simulink model "waffle_kin_sim"  (R2020a)
settings: Solver=FixedStepAuto  StartTime=0.0  StopTime=inf  FixedStep=1e-4  RelTol=1e-3
model workspace (MAT data in the model file):
  d = 0.288
  r = 0.033
undefined symbols (not defined in the file): X, Y
libraries: robotlib x11

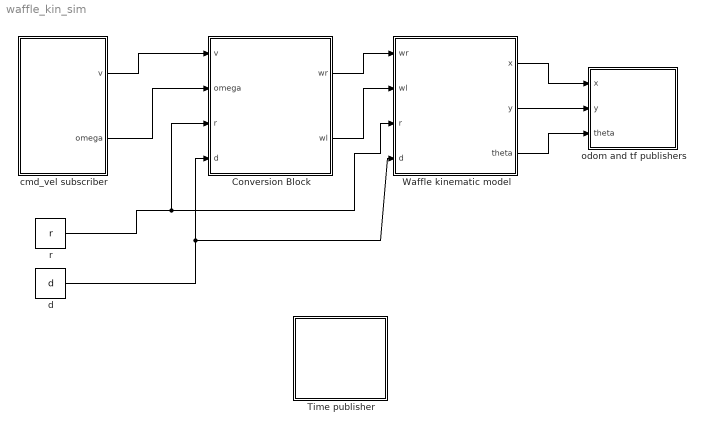
== system waffle_kin_sim ==
  Conversion Block : Subsystem  mask{state0=[0,0,0,0]}
      mask prompts: state0 "Initial conditions (x0, y0, theta0)"
  Time publisher : Subsystem
  Waffle kinematic model : Subsystem  mask{state0=[0,0,0]}
      mask prompts: state0 "Initial conditions (x0, y0, theta0)"
  cmd_vel subscriber : Subsystem
  d : Constant  Value=d
  odom and tf publishers : Subsystem  mask{simPublishRate=100}
      mask prompts: simPublishRate "Publising rate [Hz]"
  r : Constant  Value=r
  wires:
  Waffle kinematic model/1(x) -> odom and tf publishers/1(x)
  Waffle kinematic model/2(y) -> odom and tf publishers/2(y)
  Waffle kinematic model/3(theta) -> odom and tf publishers/3(theta)
  cmd_vel subscriber/1(v) -> Conversion Block/1(v)
  cmd_vel subscriber/2(omega) -> Conversion Block/2(omega)
  Conversion Block/1(wr) -> Waffle kinematic model/1(wr)
  Conversion Block/2(wl) -> Waffle kinematic model/2(wl)
  d/1 -> Conversion Block/4(d), Waffle kinematic model/4(d)
  r/1 -> Waffle kinematic model/3(r), Conversion Block/3(r)

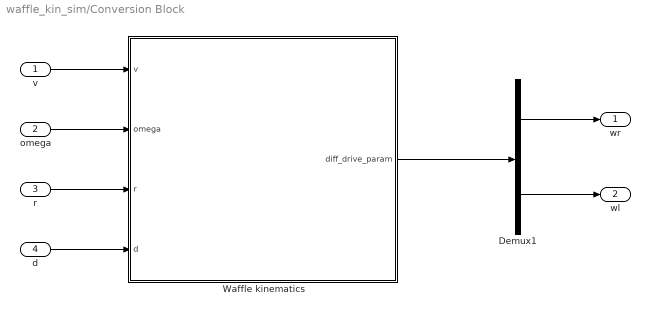
== system waffle_kin_sim/Conversion Block ==
  v : Inport
  omega : Inport  Port=2
  r : Inport  Port=3
  d : Inport  Port=4
  Demux1 : Demux  Outputs=2
  Waffle kinematics : MATLAB Function  TreatAsAtomicUnit=on
  wr : Outport  VectorParamsAs1DForOutWhenUnconnected=off
  wl : Outport  Port=2  VectorParamsAs1DForOutWhenUnconnected=off
  wires:
  Demux1/2 -> wl/1
  Demux1/1 -> wr/1
  d/1 -> Waffle kinematics/4(d)
  r/1 -> Waffle kinematics/3(r)
  v/1 -> Waffle kinematics/1(v)
  Waffle kinematics/1(diff_drive_param) -> Demux1/1
  omega/1 -> Waffle kinematics/2(omega)

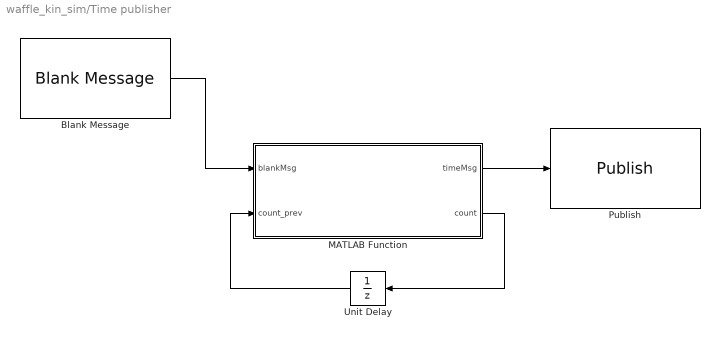
== system waffle_kin_sim/Time publisher ==
  Blank Message : robotlib/Blank Message  messageClass=Message  entityType=rosgraph_msgs/Clock  messageType=rosgraph_msgs/Clock  SampleTime=1e-4
  MATLAB Function : MATLAB Function  TreatAsAtomicUnit=on
  Publish : robotlib/Publish  topicSource=Specify your own  topic=/clock  messageType=rosgraph_msgs/Clock  messageQueueLength=1
  Unit Delay : UnitDelay  SampleTime=1e-4  HasFrameUpgradeWarning=on
  wires:
  MATLAB Function/1(timeMsg) -> Publish/1
  Blank Message/1 -> MATLAB Function/1(blankMsg)
  MATLAB Function/2(count) -> Unit Delay/1
  Unit Delay/1 -> MATLAB Function/2(count_prev)

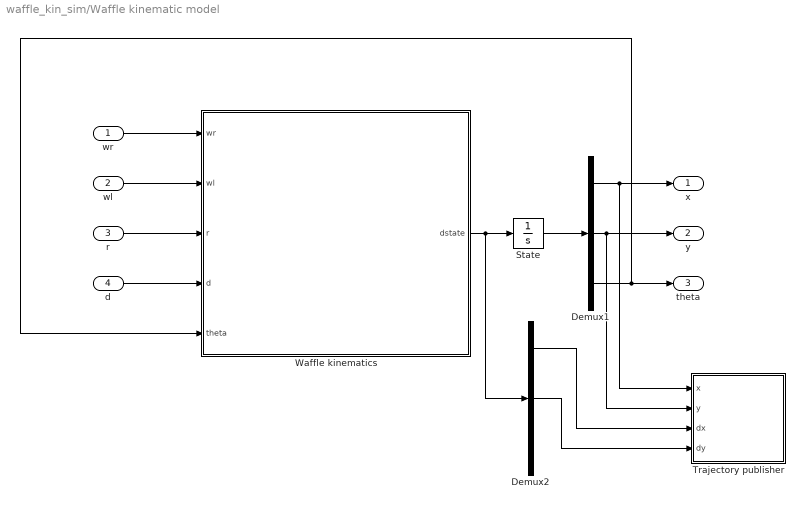
== system waffle_kin_sim/Waffle kinematic model ==
  wr : Inport
  wl : Inport  Port=2
  r : Inport  Port=3
  d : Inport  Port=4
  Demux1 : Demux  Outputs=3
  Demux2 : Demux  Outputs=3
  State : Integrator  InitialCondition=state0
  Trajectory publisher : Subsystem  mask{simPublishRate=10}
      mask prompts: simPublishRate "Publising rate [Hz]"
  Waffle kinematics : MATLAB Function  TreatAsAtomicUnit=on
  x : Outport  VectorParamsAs1DForOutWhenUnconnected=off
  y : Outport  Port=2  VectorParamsAs1DForOutWhenUnconnected=off
  theta : Outport  Port=3  VectorParamsAs1DForOutWhenUnconnected=off
  wires:
  Waffle kinematics/1(dstate) -> Demux2/1, State/1
  State/1 -> Demux1/1
  Demux1/2 -> Trajectory publisher/2(y), y/1
  Demux1/1 -> Trajectory publisher/1(x), x/1
  d/1 -> Waffle kinematics/4(d)
  r/1 -> Waffle kinematics/3(r)
  wr/1 -> Waffle kinematics/1(wr)
  wl/1 -> Waffle kinematics/2(wl)
  Demux1/3 -> Waffle kinematics/5(theta), theta/1
  Demux2/2 -> Trajectory publisher/4(dy)
  Demux2/1 -> Trajectory publisher/3(dx)

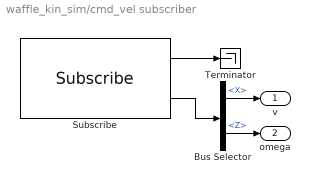
== system waffle_kin_sim/cmd_vel subscriber ==
  Bus Selector : BusSelector  OutputSignals=Linear.X,Angular.Z
  Subscribe : robotlib/Subscribe  topicSource=Specify your own  topic=/cmd_vel  messageType=geometry_msgs/Twist  sampleTime=-1  messageQueueLength=1
  Terminator : Terminator
  v : Outport
  omega : Outport  Port=2
  wires:
  Bus Selector/1 -> v/1  "<X>"
  Subscribe/2 -> Bus Selector/1
  Subscribe/1 -> Terminator/1
  Bus Selector/2 -> omega/1  "<Z>"

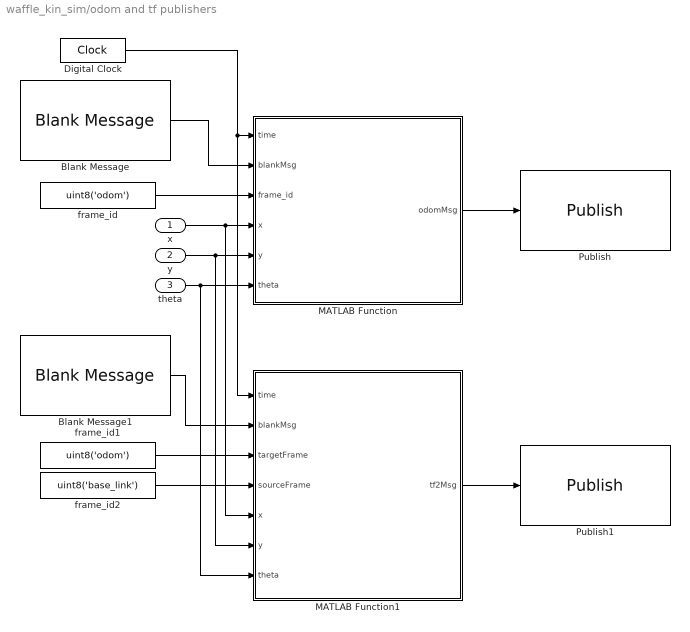
== system waffle_kin_sim/odom and tf publishers ==
  x : Inport  SampleTime=1/simPublishRate
  y : Inport  Port=2  SampleTime=1/simPublishRate
  theta : Inport  Port=3  SampleTime=1/simPublishRate
  Blank Message : robotlib/Blank Message  messageClass=Message  entityType=nav_msgs/Odometry  messageType=nav_msgs/Odometry  SampleTime=1/simPublishRate
  Blank Message1 : robotlib/Blank Message  messageClass=Message  entityType=tf2_msgs/TFMessage  messageType=tf2_msgs/TFMessage  SampleTime=1/simPublishRate
  Digital Clock : DigitalClock  SampleTime=1/simPublishRate
  MATLAB Function : MATLAB Function  TreatAsAtomicUnit=on
  MATLAB Function1 : MATLAB Function  TreatAsAtomicUnit=on
  Publish : robotlib/Publish  topicSource=Specify your own  topic=/odom  messageType=nav_msgs/Odometry  messageQueueLength=1
  Publish1 : robotlib/Publish  topicSource=Specify your own  topic=/tf  messageType=tf2_msgs/TFMessage  messageQueueLength=1
  frame_id : Constant  Value=uint8('odom')
  frame_id1 : Constant  Value=uint8('odom')
  frame_id2 : Constant  Value=uint8('base_link')
  wires:
  MATLAB Function/1(odomMsg) -> Publish/1
  theta/1 -> MATLAB Function1/7(theta), MATLAB Function/6(theta)
  y/1 -> MATLAB Function/5(y), MATLAB Function1/6(y)
  x/1 -> MATLAB Function/4(x), MATLAB Function1/5(x)
  Blank Message/1 -> MATLAB Function/2(blankMsg)
  Digital Clock/1 -> MATLAB Function1/1(time), MATLAB Function/1(time)
  frame_id/1 -> MATLAB Function/3(frame_id)
  MATLAB Function1/1(tf2Msg) -> Publish1/1
  Blank Message1/1 -> MATLAB Function1/2(blankMsg)
  frame_id1/1 -> MATLAB Function1/3(targetFrame)
  frame_id2/1 -> MATLAB Function1/4(sourceFrame)

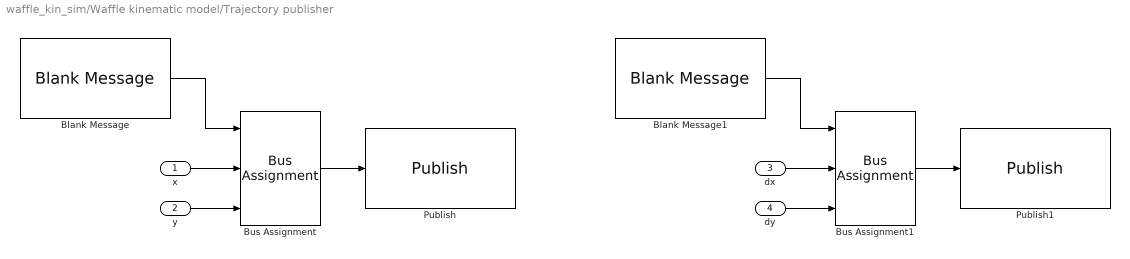
== system waffle_kin_sim/Waffle kinematic model/Trajectory publisher ==
  x : Inport  SampleTime=1/simPublishRate
  y : Inport  Port=2  SampleTime=1/simPublishRate
  dx : Inport  Port=3  SampleTime=1/simPublishRate
  dy : Inport  Port=4  SampleTime=1/simPublishRate
  Blank Message : robotlib/Blank Message  messageClass=Message  entityType=geometry_msgs/Point  messageType=geometry_msgs/Point  SampleTime=1/simPublishRate
  Blank Message1 : robotlib/Blank Message  messageClass=Message  entityType=geometry_msgs/Point  messageType=geometry_msgs/Point  SampleTime=1/simPublishRate
  Bus Assignment : BusAssignment  AssignedSignals=X,Y
  Bus Assignment1 : BusAssignment  AssignedSignals=X,Y
  Publish : robotlib/Publish  topicSource=Specify your own  topic=/actual_position  messageType=geometry_msgs/Point  messageQueueLength=1
  Publish1 : robotlib/Publish  topicSource=Specify your own  topic=/actual_velocity  messageType=geometry_msgs/Point  messageQueueLength=1
  wires:
  Bus Assignment/1 -> Publish/1
  Blank Message/1 -> Bus Assignment/1
  x/1 -> Bus Assignment/2
  y/1 -> Bus Assignment/3
  dy/1 -> Bus Assignment1/3
  dx/1 -> Bus Assignment1/2
  Blank Message1/1 -> Bus Assignment1/1
  Bus Assignment1/1 -> Publish1/1

== matlab function waffle_kin_sim/Time publisher/MATLAB Function ==
function [timeMsg,count] = generate_time_msg(blankMsg,count_prev)

time = count_prev*1e5;

blankMsg.Clock_.Sec = round(time*1e-9);
blankMsg.Clock_.Nsec = round(time-round(time));

count = count_prev+1;

timeMsg = blankMsg;

== matlab function waffle_kin_sim/odom and tf publishers/MATLAB Function1 ==
function tf2Msg = generate_tf2_msg(time,blankMsg, targetFrame, sourceFrame, x, y, theta)

% Set the number of transforms
blankMsg.Transforms_SL_Info.CurrentLength = uint32(1);

% Writing transform header
blankMsg.Transforms(1).Header.Stamp.Sec = fix(time);
blankMsg.Transforms(1).Header.Stamp.Nsec = fix((time-fix(time))*1e9);
blankMsg.Transforms(1).Header.FrameId(1:length(targetFrame)) = targetFrame;
blankMsg.Transforms(1).Header.FrameId_SL_Info.CurrentLength = uint32(length(targetFrame));

blankMsg.Transforms(1).ChildFrameId(1:length(sourceFrame)) = sourceFrame;
blankMsg.Transforms(1).ChildFrameId_SL_Info.CurrentLength = uint32(length(sourceFrame));

% Writing transform traslation and rotation data
blankMsg.Transforms(1).Transform.Translation.X = x;
blankMsg.Transforms(1).Transform.Translation.Y = y;
blankMsg.Transforms(1).Transform.Translation.Z = 0;

rotation = eul2quat([0, 0, theta], 'ZYX');
blankMsg.Transforms(1).Transform.Rotation.X = rotation(1);
blankMsg.Transforms(1).Transform.Rotation.Y = rotation(2);
blankMsg.Transforms(1).Transform.Rotation.Z = rotation(3);
blankMsg.Transforms(1).Transform.Rotation.W = rotation(4);

tf2Msg = blankMsg;

== matlab function waffle_kin_sim/Waffle kinematic model/Waffle kinematics ==
function dstate = waffle_kinematics(wr, wl, r, d, theta)

v = r*(wr+wl)/2;
omega = r*(wr-wl)/d;

dx     = v*cos(theta);
dy     = v*sin(theta);
dtheta = omega;

dstate = [dx, dy, dtheta];

== matlab function waffle_kin_sim/odom and tf publishers/MATLAB Function ==
function odomMsg = generate_odom_msg(time,blankMsg,frame_id,x,y,theta)

% Writing the message header
blankMsg.Header.Stamp.Sec = fix(time);
blankMsg.Header.Stamp.Nsec = fix((time-fix(time))*1e9);
blankMsg.Header.FrameId(1:length(frame_id)) = frame_id;
blankMsg.Header.FrameId_SL_Info.CurrentLength = uint32(length(frame_id));

% Write pose data
blankMsg.Pose.Pose.Position.X = x;
blankMsg.Pose.Pose.Position.Y = y;
blankMsg.Pose.Pose.Position.Z = 0;

orientation = eul2quat([0, 0, theta], 'ZYX');
blankMsg.Pose.Pose.Orientation.X = orientation(1);
blankMsg.Pose.Pose.Orientation.Y = orientation(2);
blankMsg.Pose.Pose.Orientation.Z = orientation(3);
blankMsg.Pose.Pose.Orientation.W = orientation(4);

odomMsg = blankMsg;

== matlab function waffle_kin_sim/Conversion Block/Waffle kinematics ==
function diff_drive_param = conversion_block(v, omega, r, d)

wr = (2*v+omega*d)/(2*r);
wl = (2*v-omega*d)/(2*r);

diff_drive_param = [wr, wl];
